simulink library "Matrix88"  (Simulink 6.2)
settings Model: LastModifiedBy=rolf

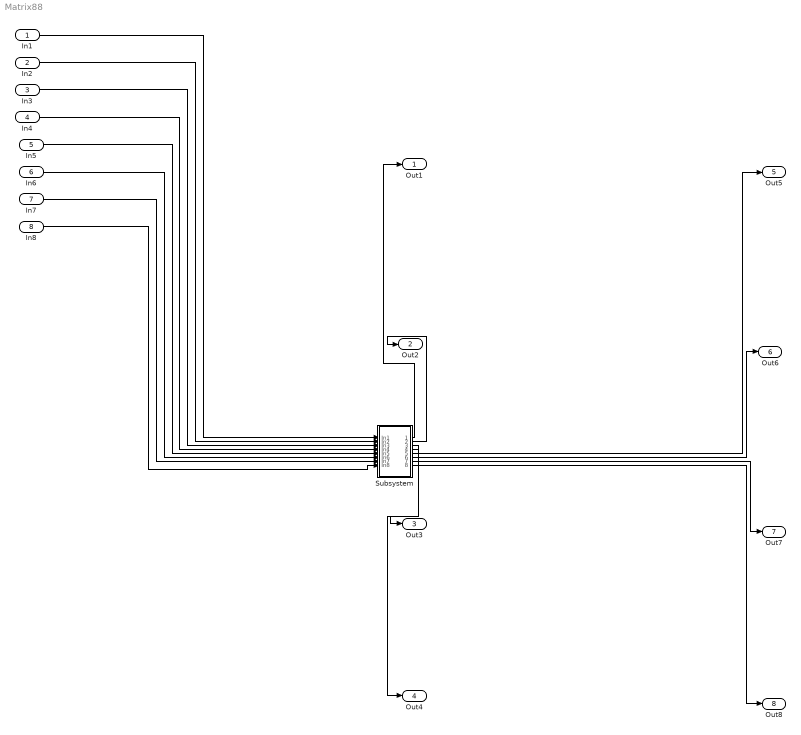
== system Matrix88 ==
  In1 : Inport  Port=1  LatchInput=off
  In2 : Inport  Port=2  LatchInput=off
  In3 : Inport  Port=3  LatchInput=off
  In4 : Inport  Port=4  LatchInput=off
  In5 : Inport  Port=5  LatchInput=off
  In6 : Inport  Port=6  LatchInput=off
  In7 : Inport  Port=7  LatchInput=off
  In8 : Inport  Port=8  LatchInput=off
  Subsystem : Subsystem
  Out1 : Outport
  Out2 : Outport  Port=2
  Out3 : Outport  Port=3
  Out4 : Outport  Port=4
  Out5 : Outport  Port=5
  Out6 : Outport  Port=6
  Out7 : Outport  Port=7
  Out8 : Outport  Port=8
  wires:
  In1/1 -> Subsystem/1(In1)
  In2/1 -> Subsystem/2(In2)
  In3/1 -> Subsystem/3(In3)
  In4/1 -> Subsystem/4(In4)
  In5/1 -> Subsystem/5(In5)
  Subsystem/1(Out1) -> Out1/1
  In6/1 -> Subsystem/6(In6)
  In7/1 -> Subsystem/7(In7)
  In8/1 -> Subsystem/8(In8)
  Subsystem/2(Out2) -> Out2/1
  Subsystem/3(Out3) -> Out3/1
  Subsystem/4(Out4) -> Out4/1
  Subsystem/5(Out5) -> Out5/1
  Subsystem/6(Out6) -> Out6/1
  Subsystem/7(Out7) -> Out7/1
  Subsystem/8(Out8) -> Out8/1

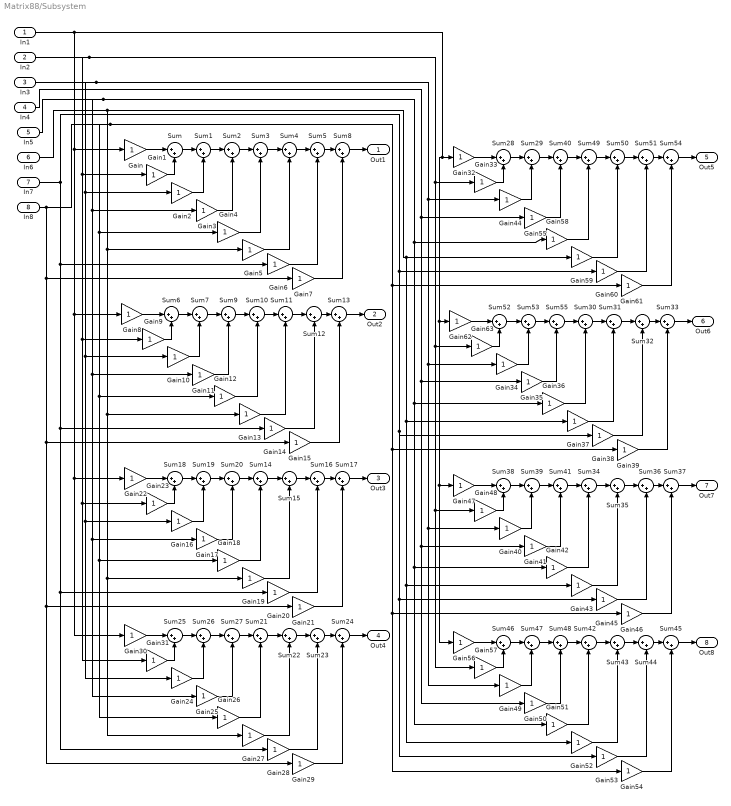
== system Matrix88/Subsystem ==
  In1 : Inport  Port=1  LatchInput=off
  In2 : Inport  Port=2  LatchInput=off
  In3 : Inport  Port=3  LatchInput=off
  In4 : Inport  Port=4  LatchInput=off
  In5 : Inport  Port=5  LatchInput=off
  In6 : Inport  Port=6  LatchInput=off
  In7 : Inport  Port=7  LatchInput=off
  In8 : Inport  Port=8  LatchInput=off
  Gain{,1..63} (64 alike) : Gain
  Sum{,1..55} (56 alike) : Sum  Inputs=|++
  Out1 : Outport
  Out2 : Outport  Port=2
  Out3 : Outport  Port=3
  Out4 : Outport  Port=4
  Out5 : Outport  Port=5
  Out6 : Outport  Port=6
  Out7 : Outport  Port=7
  Out8 : Outport  Port=8
  wires:
  Gain1/1 -> Sum/2
  Gain/1 -> Sum/1
  Sum/1 -> Sum1/1
  Gain2/1 -> Sum1/2
  Sum1/1 -> Sum2/1
  Gain3/1 -> Sum2/2
  Sum2/1 -> Sum3/1
  Sum3/1 -> Sum4/1
  Sum4/1 -> Sum5/1
  Sum5/1 -> Sum8/1
  Gain4/1 -> Sum3/2
  Gain5/1 -> Sum4/2
  Gain6/1 -> Sum5/2
  Gain7/1 -> Sum8/2
  Sum8/1 -> Out1/1
  Gain9/1 -> Sum6/2
  Gain8/1 -> Sum6/1
  Sum6/1 -> Sum7/1
  Gain10/1 -> Sum7/2
  Sum7/1 -> Sum9/1
  Gain11/1 -> Sum9/2
  Sum9/1 -> Sum10/1
  Sum10/1 -> Sum11/1
  Sum11/1 -> Sum12/1
  Sum12/1 -> Sum13/1
  Gain12/1 -> Sum10/2
  Gain13/1 -> Sum11/2
  Gain14/1 -> Sum12/2
  Gain15/1 -> Sum13/2
  Sum13/1 -> Out2/1
  Gain23/1 -> Sum18/2
  Gain22/1 -> Sum18/1
  Sum18/1 -> Sum19/1
  Gain16/1 -> Sum19/2
  Sum19/1 -> Sum20/1
  Gain17/1 -> Sum20/2
  Sum20/1 -> Sum14/1
  Sum14/1 -> Sum15/1
  Sum15/1 -> Sum16/1
  Sum16/1 -> Sum17/1
  Gain18/1 -> Sum14/2
  Gain19/1 -> Sum15/2
  Gain20/1 -> Sum16/2
  Gain21/1 -> Sum17/2
  Sum17/1 -> Out3/1
  Gain31/1 -> Sum25/2
  Gain30/1 -> Sum25/1
  Sum25/1 -> Sum26/1
  Gain24/1 -> Sum26/2
  Sum26/1 -> Sum27/1
  Gain25/1 -> Sum27/2
  Sum27/1 -> Sum21/1
  Sum21/1 -> Sum22/1
  Sum22/1 -> Sum23/1
  Sum23/1 -> Sum24/1
  Gain26/1 -> Sum21/2
  Gain27/1 -> Sum22/2
  Gain28/1 -> Sum23/2
  Gain29/1 -> Sum24/2
  Sum24/1 -> Out4/1
  Gain33/1 -> Sum28/2
  Gain32/1 -> Sum28/1
  Sum28/1 -> Sum29/1
  Gain44/1 -> Sum29/2
  Sum29/1 -> Sum40/1
  Gain55/1 -> Sum40/2
  Sum40/1 -> Sum49/1
  Sum49/1 -> Sum50/1
  Sum50/1 -> Sum51/1
  Sum51/1 -> Sum54/1
  Gain58/1 -> Sum49/2
  Gain59/1 -> Sum50/2
  Gain60/1 -> Sum51/2
  Gain61/1 -> Sum54/2
  Sum54/1 -> Out5/1
  Gain63/1 -> Sum52/2
  Gain62/1 -> Sum52/1
  Sum52/1 -> Sum53/1
  Gain34/1 -> Sum53/2
  Sum53/1 -> Sum55/1
  Gain35/1 -> Sum55/2
  Sum55/1 -> Sum30/1
  Sum30/1 -> Sum31/1
  Sum31/1 -> Sum32/1
  Sum32/1 -> Sum33/1
  Gain36/1 -> Sum30/2
  Gain37/1 -> Sum31/2
  Gain38/1 -> Sum32/2
  Gain39/1 -> Sum33/2
  Sum33/1 -> Out6/1
  Gain48/1 -> Sum38/2
  Gain47/1 -> Sum38/1
  Sum38/1 -> Sum39/1
  Gain40/1 -> Sum39/2
  Sum39/1 -> Sum41/1
  Gain41/1 -> Sum41/2
  Sum41/1 -> Sum34/1
  Sum34/1 -> Sum35/1
  Sum35/1 -> Sum36/1
  Sum36/1 -> Sum37/1
  Gain42/1 -> Sum34/2
  Gain43/1 -> Sum35/2
  Gain45/1 -> Sum36/2
  Gain46/1 -> Sum37/2
  Sum37/1 -> Out7/1
  Gain57/1 -> Sum46/2
  Gain56/1 -> Sum46/1
  Sum46/1 -> Sum47/1
  Gain49/1 -> Sum47/2
  Sum47/1 -> Sum48/1
  Gain50/1 -> Sum48/2
  Sum48/1 -> Sum42/1
  Sum42/1 -> Sum43/1
  Sum43/1 -> Sum44/1
  Sum44/1 -> Sum45/1
  Gain51/1 -> Sum42/2
  Gain52/1 -> Sum43/2
  Gain53/1 -> Sum44/2
  Gain54/1 -> Sum45/2
  Sum45/1 -> Out8/1
  In1/1 -> Gain/1, Gain8/1, Gain22/1, Gain30/1, Gain32/1, Gain62/1, Gain47/1, Gain56/1
  In2/1 -> Gain33/1, Gain63/1, Gain48/1, Gain57/1, Gain1/1, Gain9/1, Gain23/1, Gain31/1
  In3/1 -> Gain44/1, Gain34/1, Gain40/1, Gain49/1, Gain2/1, Gain10/1, Gain16/1, Gain24/1
  In4/1 -> Gain55/1, Gain35/1, Gain41/1, Gain50/1
  In5/1 -> Gain58/1, Gain36/1, Gain42/1, Gain51/1, Gain3/1, Gain11/1, Gain17/1, Gain25/1
  In6/1 -> Gain59/1, Gain37/1, Gain43/1, Gain52/1, Gain5/1, Gain13/1, Gain19/1, Gain27/1
  In7/1 -> Gain60/1, Gain38/1, Gain45/1, Gain53/1, Gain6/1, Gain14/1, Gain20/1, Gain28/1
  In8/1 -> Gain61/1, Gain39/1, Gain46/1, Gain54/1, Gain4/1, Gain12/1, Gain18/1, Gain26/1, Gain7/1, Gain15/1, Gain21/1, Gain29/1
